simulink model "probandoJoystick"  (R2017a)
settings: Solver=VariableStepAuto  StartTime=0.0  StopTime=inf  RelTol=1e-3
libraries: vrlib x1
settings Model: Creator=yellow submarine  LastModifiedBy=yellow submarine

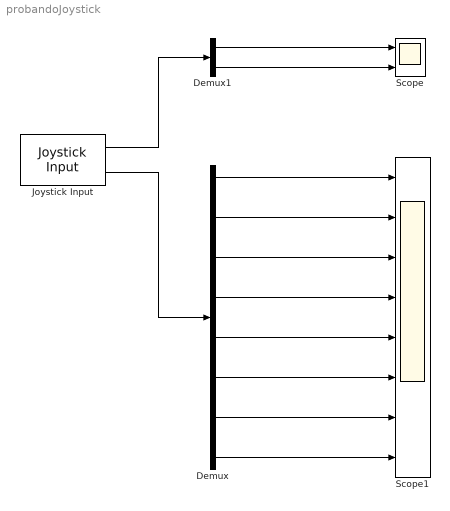
== system probandoJoystick ==
  Demux : Demux  Outputs=8
  Demux1 : Demux  Outputs=2
  Joystick Input : vrlib/Joystick Input  joyid=1  adjustports=on  forcefeed=off
      settings: SourceProductBaseCode=VR
  Scope : Scope  NumInputPorts=2
  Scope1 : Scope  NumInputPorts=8
  wires:
  Joystick Input/1 -> Demux1/1
  Demux/1 -> Scope1/1
  Joystick Input/2 -> Demux/1
  Demux/8 -> Scope1/8
  Demux/7 -> Scope1/7
  Demux/5 -> Scope1/5
  Demux/6 -> Scope1/6
  Demux/4 -> Scope1/4
  Demux/2 -> Scope1/2
  Demux/3 -> Scope1/3
  Demux1/2 -> Scope/2
  Demux1/1 -> Scope/1
